simulink model "pd_regler_simulink"  (R2025b)
settings: Solver=VariableStepAuto  StartTime=0.0  StopTime=10.0  MaxStep=1e-4  RelTol=1e-3
values from neighbouring files (symbols this model uses):
  ci = 0.01    [params.m]
  cy = 1    [params.m]
  integrator_sat_lower = -5e-2    (= -0.05)    [params.m]
  integrator_sat_upper = 5e-3    (= 0.005)    [params.m]
  jump_end_val = 0    [p_regler.m]    (also in pd_regler.m; regelstrecke.m = 1)
  jump_init_val = 0    [p_regler.m]    (also in pd_regler.m; regelstrecke.m)
  jump_time = 0    [p_regler.m]    (also in pd_regler.m; regelstrecke.m)
  K_R = K_Rs(i)    [p_regler.m]    (also in params.m = 4000)
  L = 0.1    [params.m]
  m = 10e-3    (= 0.01)    [params.m]
  R = 5    [params.m]
  sat_lower_limit = -6    [params.m]
  sat_upper_limit = 6    [params.m]
  T_V = T_Vs(i)    [pd_regler.m]
  y0 = -1e-3    (= -0.001)    [params.m]
settings Model: Creator=rishabh  LastModifiedBy=rishabh

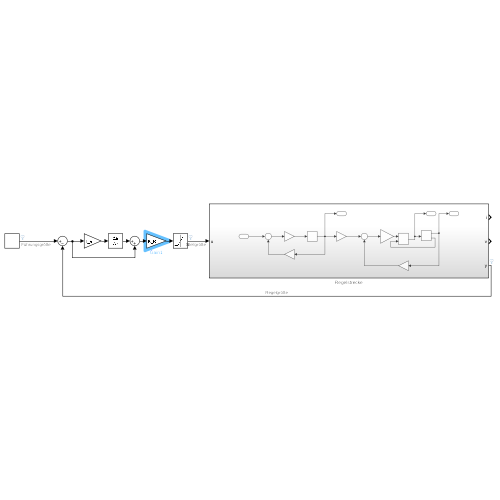
[thumbnail: Simulink's stored preview of the top-level diagram]
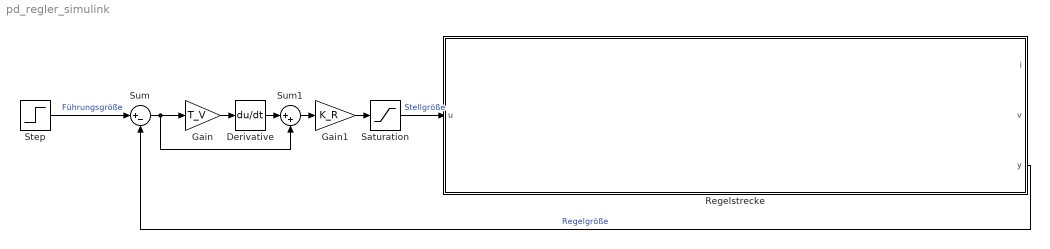
== system pd_regler_simulink ==
  Derivative : Derivative
  Gain : Gain  Gain=T_V
  Gain1 : Gain  Gain=K_R
  Regelstrecke : Subsystem
  Saturation : Saturate  UpperLimit=sat_upper_limit  LowerLimit=sat_lower_limit
  Step : Step  Time=jump_time  Before=jump_init_val  After=jump_end_val  SampleTime=0
  Sum : Sum  Inputs=|+-
  Sum1 : Sum  Inputs=|++
  wires:
  Gain1/1 -> Saturation/1
  Saturation/1 -> Regelstrecke/1(u)  "Stellgröße"
  Sum/1 -> Sum1/2, Gain/1
  Regelstrecke/3(y) -> Sum/2  "Regelgröße"
  Step/1 -> Sum/1  "Führungsgröße"
  Gain/1 -> Derivative/1
  Sum1/1 -> Gain1/1
  Derivative/1 -> Sum1/1

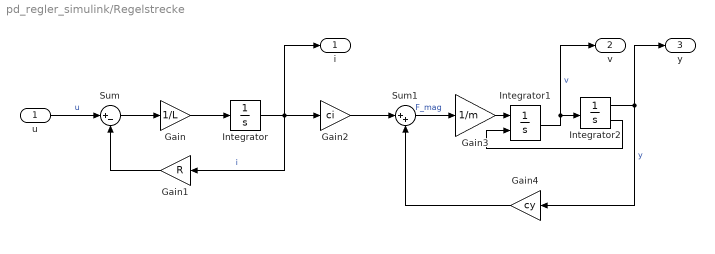
== system pd_regler_simulink/Regelstrecke ==
  u : Inport
  Gain : Gain  Gain=1/L
  Gain1 : Gain  Gain=R
  Gain2 : Gain  Gain=ci
  Gain3 : Gain  Gain=1/m
  Gain4 : Gain  Gain=cy
  Integrator : Integrator
  Integrator1 : Integrator  ExternalReset=either
  Integrator2 : Integrator  InitialCondition=y0  LimitOutput=on  UpperSaturationLimit=integrator_sat_upper  LowerSaturationLimit=integrator_sat_lower  ShowSaturationPort=on
  Sum : Sum  Inputs=|+-
  Sum1 : Sum  Inputs=|++
  i : Outport
  v : Outport  Port=2
  y : Outport  Port=3
  wires:
  Gain1/1 -> Sum/2
  Sum/1 -> Gain/1
  Gain2/1 -> Sum1/1
  Gain/1 -> Integrator/1
  Gain3/1 -> Integrator1/1
  Integrator2/1 -> Gain4/1, y/1  "y"
  u/1 -> Sum/1  "u"
  Gain4/1 -> Sum1/2
  Integrator/1 -> i/1, Gain2/1, Gain1/1  "i"
  Sum1/1 -> Gain3/1  "F_mag"
  Integrator1/1 -> v/1, Integrator2/1  "v"
  Integrator2/2 -> Integrator1/2
